simulink model "KHCN02"  (Simulink 9.1)
settings: Solver=ode45  StartTime=0.0  StopTime=12000  RelTol=1e-3  EnableMultiTasking=on
libraries: simulink x4
settings Model: Creator=Thu Ha  LastModifiedBy=Asus
settings DataIOCC: LimitDataPoints=on  SignalLoggingSaveFormat=ModelDataLogs
settings OptimizationCC: ExpressionDepthLimit=2147483647
settings DebuggingCC: SolverPrmCheckMsg=warning  FcnCallInpInsideContextMsg=warning  StateNameClashWarn=warning
settings GRTTargetCC: GeneratePreprocessorConditionals=Disable all

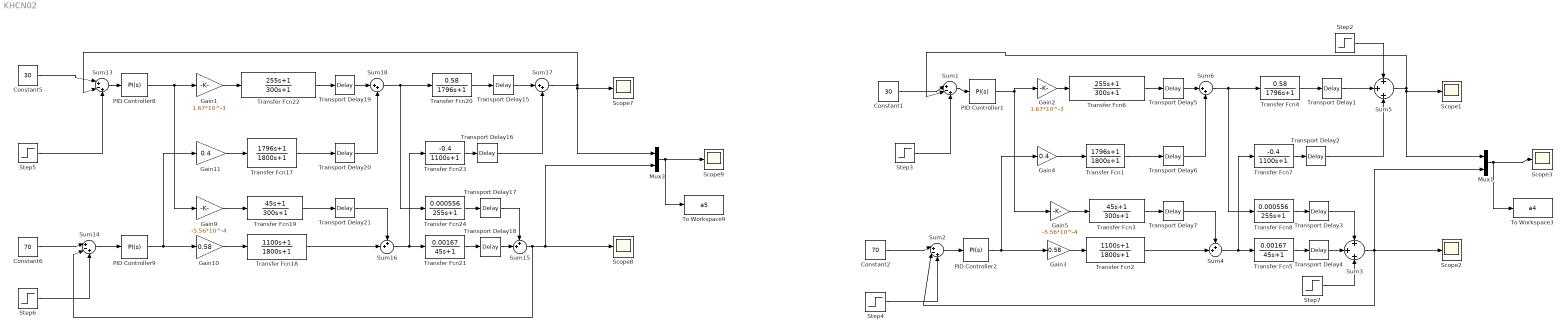
== system KHCN02 ==
  Constant1 : Constant  Value=30
  Constant2 : Constant  Value=70
  Constant5 : Constant  Value=30
  Constant6 : Constant  Value=70
  Gain1 : Gain  Gain=1.67*10^-3
  Gain10 : Gain  Gain=0.58
  Gain11 : Gain  Gain=0.4
  Gain2 : Gain  Gain=1.67*10^-3
  Gain3 : Gain  Gain=0.58
  Gain4 : Gain  Gain=0.4
  Gain5 : Gain  Gain=-5.56*10^-4
  Gain9 : Gain  Gain=-5.56*10^-4
  Mux1 : Mux  Inputs=2
  Mux3 : Mux  Inputs=2
  PID Controller1 : simulink/Continuous/PID Controller  Controller=PI  TimeDomain=Continuous-time  SampleTime=-1  IntegratorMethod=Forward Euler  FilterMethod=Forward Euler  Form=Parallel  UseFilter=on  ControllerParametersSource=internal  P=2400  I=1.38  D=0  N=100  InitialConditionSource=internal  InitialConditionForIntegrator=0  InitialConditionForFilter=0  ExternalReset=none  LimitOutput=off  UpperSaturationLimit=inf  LowerSaturationLimit=-inf  LinearizeAsGain=off  AntiWindupMode=none  Kb=1  TrackingMode=off  Kt=1  PParamMin=[]  PParamMax=[]  IParamMin=[]  IParamMax=[]  DParamMin=[]  DParamMax=[]  NParamMin=[]  NParamMax=[]  KbParamMin=[]  KbParamMax=[]  KtParamMin=[]  KtParamMax=[]  POutMin=[]  POutMax=[]  IOutMin=[]  IOutMax=[]  DOutMin=[]  DOutMax=[]  NOutMin=[]  NOutMax=[]  KbOutMin=[]  KbOutMax=[]  KtOutMin=[]  KtOutMax=[]  IntegratorOutMin=[]  IntegratorOutMax=[]  FilterOutMin=[]  FilterOutMax=[]  SumOutMin=[]  SumOutMax=[]  SumI1OutMin=[]  SumI1OutMax=[]  SumI2OutMin=[]  SumI2OutMax=[]  SumI3OutMin=[]  SumI3OutMax=[]  SumDOutMin=[]  SumDOutMax=[]  SaturationOutMin=[]  SaturationOutMax=[]  IntegratorContinuousStateAttributes=''  IntegratorStateMustResolveToSignalObject=off  IntegratorRTWStateStorageClass=Auto  FilterContinuousStateAttributes=''  FilterStateMustResolveToSignalObject=off  FilterRTWStateStorageClass=Auto  DifferentiatorICPrevScaledInput=0  DifferentiatorOutMin=[]  DifferentiatorOutMax=[]  FilterDiffOutCoefMin=[]  FilterDiffOutCoefMax=[]  SumDenOutMin=[]  SumDenOutMax=[]  SumNumOutMin=[]  SumNumOutMax=[]  ReciprocalOutMin=[]  ReciprocalOutMax=[]  DivideOutMin=[]  DivideOutMax=[]  TunerSelectOption=Transfer Function Based (PID Tuner App)
  PID Controller2 : simulink/Continuous/PID Controller  Controller=PI  TimeDomain=Continuous-time  SampleTime=-1  IntegratorMethod=Forward Euler  FilterMethod=Forward Euler  Form=Parallel  UseFilter=on  ControllerParametersSource=internal  P=2703.51319080862  I=56.5499328559093  D=0  N=100  InitialConditionSource=internal  InitialConditionForIntegrator=0  InitialConditionForFilter=0  ExternalReset=none  LimitOutput=off  UpperSaturationLimit=inf  LowerSaturationLimit=-inf  LinearizeAsGain=off  AntiWindupMode=none  Kb=1  TrackingMode=off  Kt=1  PParamMin=[]  PParamMax=[]  IParamMin=[]  IParamMax=[]  DParamMin=[]  DParamMax=[]  NParamMin=[]  NParamMax=[]  KbParamMin=[]  KbParamMax=[]  KtParamMin=[]  KtParamMax=[]  POutMin=[]  POutMax=[]  IOutMin=[]  IOutMax=[]  DOutMin=[]  DOutMax=[]  NOutMin=[]  NOutMax=[]  KbOutMin=[]  KbOutMax=[]  KtOutMin=[]  KtOutMax=[]  IntegratorOutMin=[]  IntegratorOutMax=[]  FilterOutMin=[]  FilterOutMax=[]  SumOutMin=[]  SumOutMax=[]  SumI1OutMin=[]  SumI1OutMax=[]  SumI2OutMin=[]  SumI2OutMax=[]  SumI3OutMin=[]  SumI3OutMax=[]  SumDOutMin=[]  SumDOutMax=[]  SaturationOutMin=[]  SaturationOutMax=[]  IntegratorContinuousStateAttributes=''  IntegratorStateMustResolveToSignalObject=off  IntegratorRTWStateStorageClass=Auto  FilterContinuousStateAttributes=''  FilterStateMustResolveToSignalObject=off  FilterRTWStateStorageClass=Auto  DifferentiatorICPrevScaledInput=0  DifferentiatorOutMin=[]  DifferentiatorOutMax=[]  FilterDiffOutCoefMin=[]  FilterDiffOutCoefMax=[]  SumDenOutMin=[]  SumDenOutMax=[]  SumNumOutMin=[]  SumNumOutMax=[]  ReciprocalOutMin=[]  ReciprocalOutMax=[]  DivideOutMin=[]  DivideOutMax=[]  TunerSelectOption=Transfer Function Based (PID Tuner App)
  PID Controller8 : simulink/Continuous/PID Controller  Controller=PI  TimeDomain=Continuous-time  SampleTime=-1  IntegratorMethod=Forward Euler  FilterMethod=Forward Euler  Form=Parallel  UseFilter=on  ControllerParametersSource=internal  P=2400  I=1.38  D=0  N=100  InitialConditionSource=internal  InitialConditionForIntegrator=0  InitialConditionForFilter=0  ExternalReset=none  LimitOutput=off  UpperSaturationLimit=inf  LowerSaturationLimit=-inf  LinearizeAsGain=off  AntiWindupMode=none  Kb=1  TrackingMode=off  Kt=1  PParamMin=[]  PParamMax=[]  IParamMin=[]  IParamMax=[]  DParamMin=[]  DParamMax=[]  NParamMin=[]  NParamMax=[]  KbParamMin=[]  KbParamMax=[]  KtParamMin=[]  KtParamMax=[]  POutMin=[]  POutMax=[]  IOutMin=[]  IOutMax=[]  DOutMin=[]  DOutMax=[]  NOutMin=[]  NOutMax=[]  KbOutMin=[]  KbOutMax=[]  KtOutMin=[]  KtOutMax=[]  IntegratorOutMin=[]  IntegratorOutMax=[]  FilterOutMin=[]  FilterOutMax=[]  SumOutMin=[]  SumOutMax=[]  SumI1OutMin=[]  SumI1OutMax=[]  SumI2OutMin=[]  SumI2OutMax=[]  SumI3OutMin=[]  SumI3OutMax=[]  SumDOutMin=[]  SumDOutMax=[]  SaturationOutMin=[]  SaturationOutMax=[]  IntegratorContinuousStateAttributes=''  IntegratorStateMustResolveToSignalObject=off  IntegratorRTWStateStorageClass=Auto  FilterContinuousStateAttributes=''  FilterStateMustResolveToSignalObject=off  FilterRTWStateStorageClass=Auto  DifferentiatorICPrevScaledInput=0  DifferentiatorOutMin=[]  DifferentiatorOutMax=[]  FilterDiffOutCoefMin=[]  FilterDiffOutCoefMax=[]  SumDenOutMin=[]  SumDenOutMax=[]  SumNumOutMin=[]  SumNumOutMax=[]  ReciprocalOutMin=[]  ReciprocalOutMax=[]  DivideOutMin=[]  DivideOutMax=[]  TunerSelectOption=Transfer Function Based (PID Tuner App)
  PID Controller9 : simulink/Continuous/PID Controller  Controller=PI  TimeDomain=Continuous-time  SampleTime=-1  IntegratorMethod=Forward Euler  FilterMethod=Forward Euler  Form=Parallel  UseFilter=on  ControllerParametersSource=internal  P=2703.51319080862  I=56.5499328559093  D=0  N=100  InitialConditionSource=internal  InitialConditionForIntegrator=0  InitialConditionForFilter=0  ExternalReset=none  LimitOutput=off  UpperSaturationLimit=inf  LowerSaturationLimit=-inf  LinearizeAsGain=off  AntiWindupMode=none  Kb=1  TrackingMode=off  Kt=1  PParamMin=[]  PParamMax=[]  IParamMin=[]  IParamMax=[]  DParamMin=[]  DParamMax=[]  NParamMin=[]  NParamMax=[]  KbParamMin=[]  KbParamMax=[]  KtParamMin=[]  KtParamMax=[]  POutMin=[]  POutMax=[]  IOutMin=[]  IOutMax=[]  DOutMin=[]  DOutMax=[]  NOutMin=[]  NOutMax=[]  KbOutMin=[]  KbOutMax=[]  KtOutMin=[]  KtOutMax=[]  IntegratorOutMin=[]  IntegratorOutMax=[]  FilterOutMin=[]  FilterOutMax=[]  SumOutMin=[]  SumOutMax=[]  SumI1OutMin=[]  SumI1OutMax=[]  SumI2OutMin=[]  SumI2OutMax=[]  SumI3OutMin=[]  SumI3OutMax=[]  SumDOutMin=[]  SumDOutMax=[]  SaturationOutMin=[]  SaturationOutMax=[]  IntegratorContinuousStateAttributes=''  IntegratorStateMustResolveToSignalObject=off  IntegratorRTWStateStorageClass=Auto  FilterContinuousStateAttributes=''  FilterStateMustResolveToSignalObject=off  FilterRTWStateStorageClass=Auto  DifferentiatorICPrevScaledInput=0  DifferentiatorOutMin=[]  DifferentiatorOutMax=[]  FilterDiffOutCoefMin=[]  FilterDiffOutCoefMax=[]  SumDenOutMin=[]  SumDenOutMax=[]  SumNumOutMin=[]  SumNumOutMax=[]  ReciprocalOutMin=[]  ReciprocalOutMax=[]  DivideOutMin=[]  DivideOutMax=[]  TunerSelectOption=Transfer Function Based (PID Tuner App)
  Scope{1..3,7..9} (6 alike) : Scope
  Step2 : Step  Time=9000  After=5  SampleTime=0
  Step3 : Step  Time=6000  After=5  SampleTime=0
  Step4 : Step  Time=4000  After=5  SampleTime=0
  Step5 : Step  Time=6000  After=5  SampleTime=0
  Step6 : Step  Time=4000  After=5  SampleTime=0
  Step7 : Step  Time=5000  After=5  SampleTime=0
  Sum{1..2,13..14} (4 alike) : Sum  Inputs=|+-+  SaturateOnIntegerOverflow=on  InputSameDT=on  OutDataTypeStr=Inherit: Same as first input
  Sum15 : Sum  Inputs=++|  SaturateOnIntegerOverflow=on  InputSameDT=on  OutDataTypeStr=Inherit: Same as first input
  Sum16 : Sum  Inputs=++|  SaturateOnIntegerOverflow=on  InputSameDT=on  OutDataTypeStr=Inherit: Same as first input
  Sum17 : Sum  Inputs=|++  SaturateOnIntegerOverflow=on  InputSameDT=on  OutDataTypeStr=Inherit: Same as first input
  Sum18 : Sum  Inputs=|++  SaturateOnIntegerOverflow=on  InputSameDT=on  OutDataTypeStr=Inherit: Same as first input
  Sum3 : Sum  Inputs=+|+|+  SaturateOnIntegerOverflow=on  InputSameDT=on  OutDataTypeStr=Inherit: Same as first input
  Sum4 : Sum  Inputs=++|  SaturateOnIntegerOverflow=on  InputSameDT=on  OutDataTypeStr=Inherit: Same as first input
  Sum5 : Sum  Inputs=+|+|+  SaturateOnIntegerOverflow=on  InputSameDT=on  OutDataTypeStr=Inherit: Same as first input
  Sum6 : Sum  Inputs=|++  SaturateOnIntegerOverflow=on  InputSameDT=on  OutDataTypeStr=Inherit: Same as first input
  To Workspace3 : ToWorkspace  VariableName=a4  SampleTime=1
  To Workspace9 : ToWorkspace  VariableName=a5  SampleTime=1
  Transfer Fcn1 : TransferFcn  Numerator=[1796 1]  Denominator=[1800 1]
  Transfer Fcn17 : TransferFcn  Numerator=[1796 1]  Denominator=[1800 1]
  Transfer Fcn18 : TransferFcn  Numerator=[1100 1]  Denominator=[1800 1]
  Transfer Fcn19 : TransferFcn  Numerator=[45 1]  Denominator=[300 1]
  Transfer Fcn2 : TransferFcn  Numerator=[1100 1]  Denominator=[1800 1]
  Transfer Fcn20 : TransferFcn  Numerator=0.58  Denominator=[1796 1]
  Transfer Fcn21 : TransferFcn  Numerator=0.00167  Denominator=[45 1]
  Transfer Fcn22 : TransferFcn  Numerator=[255 1]  Denominator=[300 1]
  Transfer Fcn23 : TransferFcn  Numerator=-0.4  Denominator=[1100 1]
  Transfer Fcn24 : TransferFcn  Numerator=0.000556  Denominator=[255 1]
  Transfer Fcn3 : TransferFcn  Numerator=[45 1]  Denominator=[300 1]
  Transfer Fcn4 : TransferFcn  Numerator=0.58  Denominator=[1796 1]
  Transfer Fcn5 : TransferFcn  Numerator=0.00167  Denominator=[45 1]
  Transfer Fcn6 : TransferFcn  Numerator=[255 1]  Denominator=[300 1]
  Transfer Fcn7 : TransferFcn  Numerator=-0.4  Denominator=[1100 1]
  Transfer Fcn8 : TransferFcn  Numerator=0.000556  Denominator=[255 1]
  Transport Delay1 : TransportDelay  DelayTime=90
  Transport Delay15 : TransportDelay  DelayTime=90
  Transport Delay16 : TransportDelay  DelayTime=92
  Transport Delay17 : TransportDelay  DelayTime=0.18
  Transport Delay18 : TransportDelay  DelayTime=0.02
  Transport Delay19 : TransportDelay  DelayTime=91.72
  Transport Delay2 : TransportDelay  DelayTime=92
  Transport Delay20 : TransportDelay  DelayTime=2
  Transport Delay21 : TransportDelay  DelayTime=91.98
  Transport Delay3 : TransportDelay  DelayTime=0.18
  Transport Delay4 : TransportDelay  DelayTime=0.02
  Transport Delay5 : TransportDelay  DelayTime=91.72
  Transport Delay6 : TransportDelay  DelayTime=2
  Transport Delay7 : TransportDelay  DelayTime=91.98
  wires:
  Constant5/1 -> Sum13/1
  Sum13/1 -> PID Controller8/1
  Transfer Fcn20/1 -> Transport Delay15/1
  Constant6/1 -> Sum14/1
  Sum14/1 -> PID Controller9/1
  Transfer Fcn21/1 -> Transport Delay18/1
  Transfer Fcn23/1 -> Transport Delay16/1
  Sum15/1 -> Scope8/1, Mux3/2, Sum14/2
  Step5/1 -> Sum13/3
  Mux3/1 -> To Workspace9/1, Scope9/1
  Sum16/1 -> Transfer Fcn21/1, Transfer Fcn23/1
  Step6/1 -> Sum14/3
  Sum17/1 -> Scope7/1, Mux3/1, Sum13/2
  Transfer Fcn24/1 -> Transport Delay17/1
  Sum18/1 -> Transfer Fcn20/1, Transfer Fcn24/1
  Transport Delay19/1 -> Sum18/1
  Transfer Fcn22/1 -> Transport Delay19/1
  Transfer Fcn17/1 -> Transport Delay20/1
  Transfer Fcn18/1 -> Sum16/2
  Transfer Fcn19/1 -> Transport Delay21/1
  Gain1/1 -> Transfer Fcn22/1
  Gain11/1 -> Transfer Fcn17/1
  Gain9/1 -> Transfer Fcn19/1
  Gain10/1 -> Transfer Fcn18/1
  Transport Delay18/1 -> Sum15/2
  Transport Delay17/1 -> Sum15/1
  PID Controller9/1 -> Gain10/1, Gain11/1
  PID Controller8/1 -> Gain9/1, Gain1/1
  Transport Delay20/1 -> Sum18/2
  Transport Delay21/1 -> Sum16/1
  Constant1/1 -> Sum1/1
  Sum1/1 -> PID Controller1/1
  Transfer Fcn4/1 -> Transport Delay1/1
  Constant2/1 -> Sum2/1
  Sum2/1 -> PID Controller2/1
  Transfer Fcn5/1 -> Transport Delay4/1
  Transfer Fcn7/1 -> Transport Delay2/1
  Sum3/1 -> Scope2/1, Mux1/2, Sum2/2
  Step3/1 -> Sum1/3
  Mux1/1 -> To Workspace3/1, Scope3/1
  Sum4/1 -> Transfer Fcn5/1, Transfer Fcn7/1
  Step4/1 -> Sum2/3
  Transport Delay1/1 -> Sum5/2
  Sum5/1 -> Scope1/1, Mux1/1, Sum1/2
  Transfer Fcn8/1 -> Transport Delay3/1
  Sum6/1 -> Transfer Fcn4/1, Transfer Fcn8/1
  Transport Delay5/1 -> Sum6/1
  Transfer Fcn6/1 -> Transport Delay5/1
  Transfer Fcn1/1 -> Transport Delay6/1
  Transfer Fcn2/1 -> Sum4/2
  Transfer Fcn3/1 -> Transport Delay7/1
  Gain2/1 -> Transfer Fcn6/1
  Gain4/1 -> Transfer Fcn1/1
  Gain5/1 -> Transfer Fcn3/1
  Gain3/1 -> Transfer Fcn2/1
  Transport Delay4/1 -> Sum3/2
  Transport Delay3/1 -> Sum3/1
  PID Controller2/1 -> Gain3/1, Gain4/1
  PID Controller1/1 -> Gain2/1, Gain5/1
  Transport Delay6/1 -> Sum6/2
  Transport Delay7/1 -> Sum4/1
  Step7/1 -> Sum3/3
  Transport Delay15/1 -> Sum17/1
  Transport Delay16/1 -> Sum17/2
  Step2/1 -> Sum5/1
  Transport Delay2/1 -> Sum5/3
